simulink model "sin_str0_leaderVel_exp4"  (R2016a)
settings: Solver=FixedStepAuto  StartTime=0.0  StopTime=inf  RelTol=1e-3
undefined symbols (not defined in the file or in its folder): Angular, Linear
libraries: robotlib x2
settings Model: Creator=ece446  LastModifiedBy=ece446
settings OptimizationCC: OptimizeModelRefInitCode=on  LifeSpan=Inf  MaxStackSize=64
settings HardwareCC: ProdBitPerPointer=32  ProdLargestAtomicFloat=None  ProdIntDivRoundTo=Undefined  ProdEndianess=Unspecified  ProdWordSize=32  ProdHWDeviceType=Generic->Unspecified (assume 32-bit Generic)  UseEmbeddedCoderFeatures=off
settings RTWCC: SystemTargetFile=ert.tlc  HardwareBoard=Robot Operating System (ROS)  TemplateMakefile=ert_default_tmf  GenerateReport=on  Toolchain=Catkin  IncludeHyperlinkInReport=on  LaunchReport=on  TargetLang=C++  GenerateTraceInfo=on  GenerateTraceReport=on  GenerateTraceReportSl=on  GenerateTraceReportSf=on  GenerateTraceReportEml=on
settings CodeAppCC: ForceParamTrailComments=on  IgnoreCustomStorageClasses=off  OperatorAnnotations=on  SimulinkDataObjDesc=on  SFDataObjDesc=on  MATLABFcnDesc=on  InsertBlockDesc=on  MATLABSourceComments=on
settings ERTTargetCC: SupportNonInlinedSFcns=on

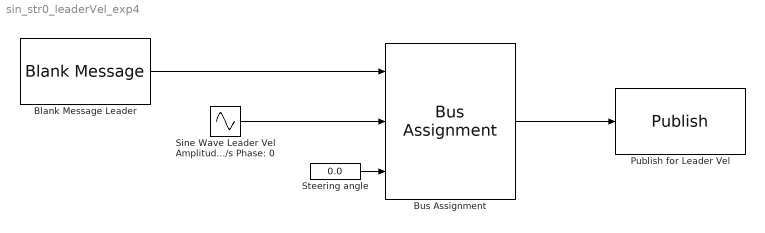
== system sin_str0_leaderVel_exp4 ==
  Blank Message Leader : robotlib/Blank Message  SourceLibraryInfo=This block requires Robotics System Toolbox  messageType=geometry_msgs/Twist  SampleTime=inf
  Bus Assignment : BusAssignment  AssignedSignals=Linear.X,Angular.Z
  Publish for Leader Vel : robotlib/Publish  SourceLibraryInfo=This block requires Robotics System Toolbox  topicSource=Select from ROS network  topic=/azcar_sim/cmd_vel  messageType=geometry_msgs/Twist  messageQueueLength=1
  "Sine Wave Leader Vel Amplitude: 1 Bias: 3 Frequency: 5/2*pi rad/s Phase: 0 " : Sin  Amplitude=5  Bias=3  Frequency=0.7958  SampleTime=0
  Steering angle : Constant  Value=0.0
  wires:
  Blank Message Leader/1 -> Bus Assignment/1
  Bus Assignment/1 -> Publish for Leader Vel/1
  "Sine Wave Leader Vel Amplitude: 1 Bias: 3 Frequency: 5/2*pi rad/s Phase: 0 "/1 -> Bus Assignment/2
  Steering angle/1 -> Bus Assignment/3
